simulink library "csu_gsh_gravity_spherical_harmonic_lib"  (R2014b)
settings: Solver=ode45  StartTime=0.0  StopTime=10.0  RelTol=1e-3
undefined symbols (not defined in the file or in its folder): central_body_flattening, gsh_a, gsh_b, gsh_c, gsh_deg, gsh_e, gsh_ep, gsh_n_degree, gsh_ord, gsh_s, magnitude
undefined symbols (not defined in the file): central_body_gravity_mu, central_body_radius
libraries: util_quat_lib x4, util_info_lib x2, util_common_lib x1
settings Model: Creator=mstewart  LastModifiedBy=mstewart

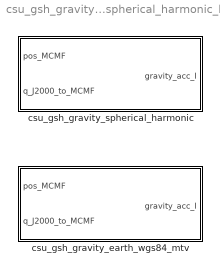
== system csu_gsh_gravity_spherical_harmonic_lib ==
  csu_gsh_gravity_earth_wgs84_mtv : Subsystem
  csu_gsh_gravity_spherical_harmonic : Subsystem  mask{mu_central_body=central_body_gravity_mu, r_central_body=central_body_radius}
      mask prompts: mu_central_body "Mu parameter for central body"; r_central_body "Radius of central body"

== system csu_gsh_gravity_spherical_harmonic_lib/csu_gsh_gravity_earth_wgs84_mtv ==
  pos_MCMF : Inport
  q_J2000_to_MCMF : Inport  Port=2
  Library Information : util_info_lib/Library Information  owner='NONE'
  earth_surface_gravity_with_j2 : Subsystem
  quaternion_conjugate : util_quat_lib/quaternion_conjugate  SystemSampleTime=-1
  quaternion_frame_transformation : util_quat_lib/quaternion_frame_transformation  SystemSampleTime=-1
  gravity_acc_I : Outport
  wires:
  earth_surface_gravity_with_j2/1(g_MCMF) -> quaternion_frame_transformation/1  "gravity_acc_MCMF"
  pos_MCMF/1 -> earth_surface_gravity_with_j2/1(pos_MCMF)
  quaternion_conjugate/1 -> quaternion_frame_transformation/2
  quaternion_frame_transformation/1 -> gravity_acc_I/1
  q_J2000_to_MCMF/1 -> quaternion_conjugate/1

== system csu_gsh_gravity_spherical_harmonic_lib/csu_gsh_gravity_spherical_harmonic ==
  pos_MCMF : Inport
  q_J2000_to_MCMF : Inport  Port=2
  Library Information : util_info_lib/Library Information  owner='NONE'
  Spherical Harmonic Gravity Model : Subsystem
      mask Display:
      | port_label('input',1,'pos\_MCMF','texmode','on')
      | port_label('output',1,'g\_MCMF','texmode','on')
      | disp('Spherical Harmonic Gravity Model')
      | color('blue')
      | text(0.05,0.02,'MoonEx',...
      |  	'HorizontalAlignment','Left',...
      | 	'VerticalAlignment','bottom')
  quaternion_conjugate : util_quat_lib/quaternion_conjugate  SystemSampleTime=-1
  quaternion_frame_transformation : util_quat_lib/quaternion_frame_transformation  SystemSampleTime=-1
  gravity_acc_I : Outport
  wires:
  Spherical Harmonic Gravity Model/1(g_MCMF) -> quaternion_frame_transformation/1  "gravity_acc_MCMF"
  pos_MCMF/1 -> Spherical Harmonic Gravity Model/1(pos_MCMF)
  quaternion_conjugate/1 -> quaternion_frame_transformation/2
  quaternion_frame_transformation/1 -> gravity_acc_I/1
  q_J2000_to_MCMF/1 -> quaternion_conjugate/1

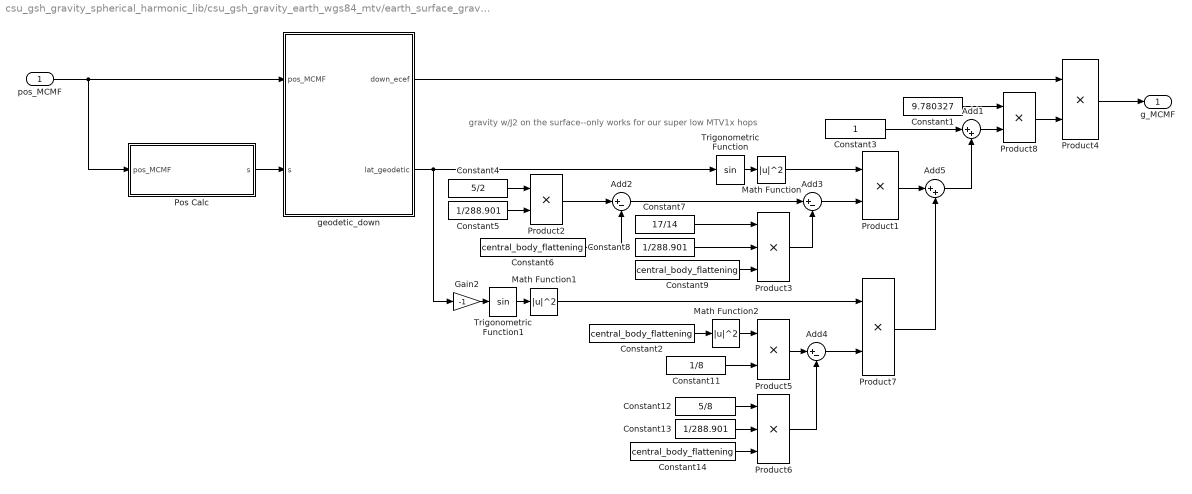
== system csu_gsh_gravity_spherical_harmonic_lib/csu_gsh_gravity_earth_wgs84_mtv/earth_surface_gravity_with_j2 ==
  note: gravity w/J2 on the surface--only works for our super low MTV1x hops
  pos_MCMF : Inport
  Add1 : Sum  Inputs=|++
  Add2 : Sum  Inputs=|+-
  Add3 : Sum  Inputs=|+-
  Add4 : Sum  Inputs=|+-
  Add5 : Sum  Inputs=|++
  Constant1 : Constant  Value=9.780327
  Constant11 : Constant  Value=1/8
  Constant12 : Constant  Value=5/8
  Constant13 : Constant  Value=1/288.901
  Constant{2,6,9,14} (4 alike) : Constant  Value=central_body_flattening
  Constant3 : Constant
  Constant4 : Constant  Value=5/2
  Constant5 : Constant  Value=1/288.901
  Constant7 : Constant  Value=17/14
  Constant8 : Constant  Value=1/288.901
  Gain2 : Gain  Gain=-1
  Math Function : Math  Operator=magnitude^2  SaturateOnIntegerOverflow=on
  Math Function1 : Math  Operator=magnitude^2  SaturateOnIntegerOverflow=on
  Math Function2 : Math  Operator=magnitude^2  SaturateOnIntegerOverflow=on
  Pos Calc : Subsystem
  Product{1..2,4..5,7..8} (6 alike) : Product
  Product3 : Product  Inputs=3
  Product6 : Product  Inputs=3
  Trigonometric Function : Trigonometry
  Trigonometric Function1 : Trigonometry
  geodetic_down : Subsystem
  g_MCMF : Outport
  wires:
  geodetic_down/1(down_ecef) -> Product4/1
  Product8/1 -> Product4/2
  Constant1/1 -> Product8/1
  Add1/1 -> Product8/2
  Add5/1 -> Add1/2
  Product7/1 -> Add5/2
  Product1/1 -> Add5/1
  Math Function1/1 -> Product7/1
  Add4/1 -> Product7/2
  Product6/1 -> Add4/2
  Product5/1 -> Add4/1
  Constant14/1 -> Product6/3
  Constant13/1 -> Product6/2
  Constant12/1 -> Product6/1
  Constant11/1 -> Product5/2
  Math Function2/1 -> Product5/1
  Constant2/1 -> Math Function2/1
  Add3/1 -> Product1/2
  Math Function/1 -> Product1/1
  Product3/1 -> Add3/2
  Add2/1 -> Add3/1
  Constant9/1 -> Product3/3
  Constant8/1 -> Product3/2
  Constant7/1 -> Product3/1
  Constant6/1 -> Add2/2
  Product2/1 -> Add2/1
  Constant5/1 -> Product2/2
  Constant4/1 -> Product2/1
  Gain2/1 -> Trigonometric Function1/1
  geodetic_down/2(lat_geodetic) -> Trigonometric Function/1, Gain2/1
  Trigonometric Function1/1 -> Math Function1/1
  Trigonometric Function/1 -> Math Function/1
  Constant3/1 -> Add1/1
  pos_MCMF/1 -> geodetic_down/1(pos_MCMF), Pos Calc/1(pos_MCMF)
  Pos Calc/1(s) -> geodetic_down/2(s)
  Product4/1 -> g_MCMF/1

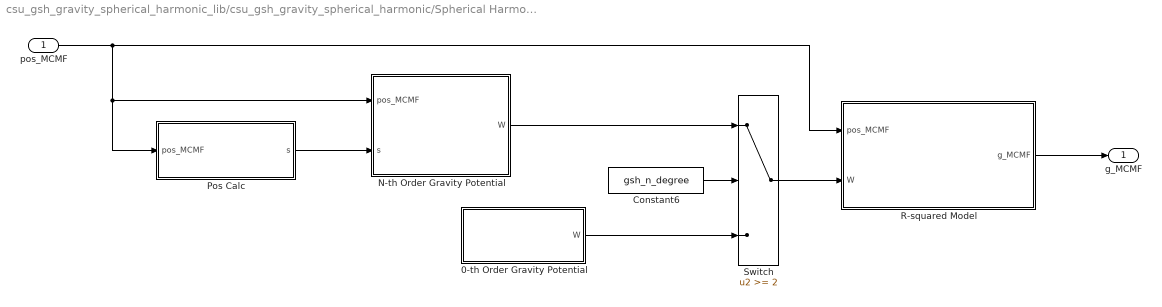
== system csu_gsh_gravity_spherical_harmonic_lib/csu_gsh_gravity_spherical_harmonic/Spherical Harmonic Gravity Model ==
  pos_MCMF : Inport
  0-th Order Gravity Potential : Subsystem
  Constant6 : Constant  Value=gsh_n_degree
  N-th Order Gravity Potential : Subsystem
  Pos Calc : Subsystem
  R-squared Model : Subsystem
  Switch : Switch  Threshold=2
  g_MCMF : Outport
  wires:
  pos_MCMF/1 -> R-squared Model/1(pos_MCMF), N-th Order Gravity Potential/1(pos_MCMF), Pos Calc/1(pos_MCMF)
  Switch/1 -> R-squared Model/2(W)
  Pos Calc/1(s) -> N-th Order Gravity Potential/2(s)
  0-th Order Gravity Potential/1(W) -> Switch/3
  N-th Order Gravity Potential/1(W) -> Switch/1
  Constant6/1 -> Switch/2
  R-squared Model/1(g_MCMF) -> g_MCMF/1

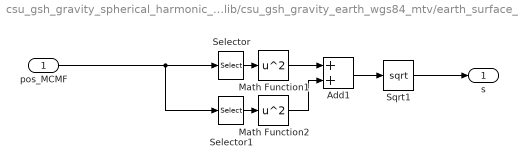
== system csu_gsh_gravity_spherical_harmonic_lib/csu_gsh_gravity_earth_wgs84_mtv/earth_surface_gravity_with_j2/Pos Calc ==
  pos_MCMF : Inport
  Add1 : Sum
  Math Function1 : Math  Operator=square  SaturateOnIntegerOverflow=on
  Math Function2 : Math  Operator=square  SaturateOnIntegerOverflow=on
  Selector : Selector  InputPortWidth=3  Indices=[1]
  Selector1 : Selector  InputPortWidth=3  Indices=[2]
  Sqrt1 : Sqrt  SaturateOnIntegerOverflow=on
  s : Outport
  wires:
  Math Function2/1 -> Add1/2
  Math Function1/1 -> Add1/1
  Sqrt1/1 -> s/1
  Add1/1 -> Sqrt1/1
  Selector1/1 -> Math Function2/1
  Selector/1 -> Math Function1/1
  pos_MCMF/1 -> Selector/1, Selector1/1

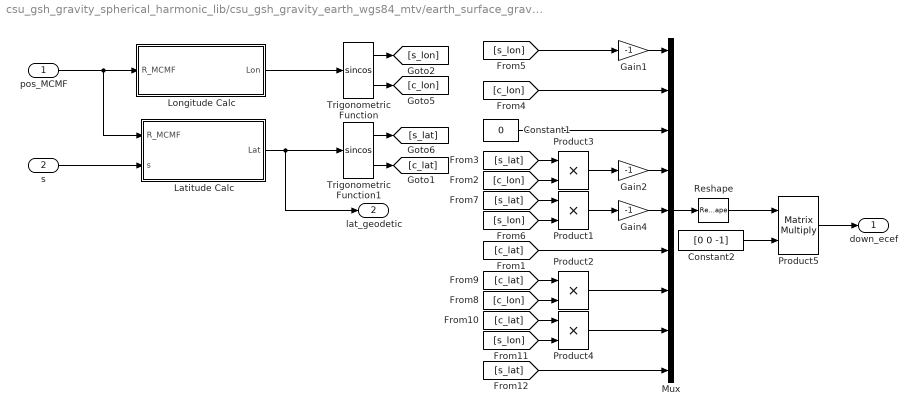
== system csu_gsh_gravity_spherical_harmonic_lib/csu_gsh_gravity_earth_wgs84_mtv/earth_surface_gravity_with_j2/geodetic_down ==
  pos_MCMF : Inport
  s : Inport  Port=2
  Constant1 : Constant  Value=0
  Constant2 : Constant  Value=[0 0 -1]
  Gain1 : Gain  Gain=-1
  Gain2 : Gain  Gain=-1
  Gain4 : Gain  Gain=-1
  Latitude Calc : Subsystem
  Longitude Calc : Subsystem
  Mux : Mux  Inputs=9
  Product{1..4} (4 alike) : Product  RndMeth=Zero
  Product5 : Product  Multiplication=Matrix(*)  RndMeth=Zero
  Reshape : Reshape  OutputDimensionality=Customize  OutputDimensions=[3,3]
  Trigonometric Function : Trigonometry  Operator=sincos
  Trigonometric Function1 : Trigonometry  Operator=sincos
  down_ecef : Outport
  lat_geodetic : Outport  Port=2
  wires:
  s/1 -> Latitude Calc/2(s)
  Product5/1 -> down_ecef/1
  Longitude Calc/1(Lon) -> Trigonometric Function/1
  Latitude Calc/1(Lat) -> Trigonometric Function1/1, lat_geodetic/1
  pos_MCMF/1 -> Longitude Calc/1(R_MCMF), Latitude Calc/1(R_MCMF)
  Trigonometric Function/1 -> [s_lon]
  Trigonometric Function/2 -> [c_lon]
  Trigonometric Function1/1 -> [s_lat]
  Trigonometric Function1/2 -> [c_lat]
  Gain1/1 -> Mux/1
  [s_lon] -> Gain1/1
  [c_lon] -> Mux/2
  Constant1/1 -> Mux/3
  [s_lat] -> Product3/1
  [c_lon] -> Product3/2
  Product3/1 -> Gain2/1
  Gain2/1 -> Mux/4
  [s_lat] -> Product1/1
  [s_lon] -> Product1/2
  Product1/1 -> Gain4/1
  Gain4/1 -> Mux/5
  [c_lat] -> Mux/6
  [c_lat] -> Product2/1
  Product2/1 -> Mux/7
  [c_lon] -> Product2/2
  [c_lat] -> Product4/1
  Product4/1 -> Mux/8
  [s_lon] -> Product4/2
  [s_lat] -> Mux/9
  Mux/1 -> Reshape/1
  Reshape/1 -> Product5/1
  Constant2/1 -> Product5/2

== system csu_gsh_gravity_spherical_harmonic_lib/csu_gsh_gravity_spherical_harmonic/Spherical Harmonic Gravity Model/0-th Order Gravity Potential ==
  Constant : Constant  Value=0
  W : Outport
  wires:
  Constant/1 -> W/1

== system csu_gsh_gravity_spherical_harmonic_lib/csu_gsh_gravity_spherical_harmonic/Spherical Harmonic Gravity Model/N-th Order Gravity Potential ==
  pos_MCMF : Inport
  s : Inport  Port=2
  Altitude Calc : Subsystem
  Gravity Potential : Subsystem
  Latitude Calc : Subsystem
  Longitude Calc : Subsystem
  W : Outport
  wires:
  s/1 -> Latitude Calc/2(s), Altitude Calc/2(s)
  Gravity Potential/1(W) -> W/1
  Longitude Calc/1(Lon) -> Gravity Potential/1(Lon)
  Altitude Calc/1(Alt) -> Gravity Potential/3(Alt)
  Latitude Calc/1(Lat) -> Altitude Calc/1(Lat), Gravity Potential/2(Lat)
  pos_MCMF/1 -> Longitude Calc/1(R_MCMF), Latitude Calc/1(R_MCMF)

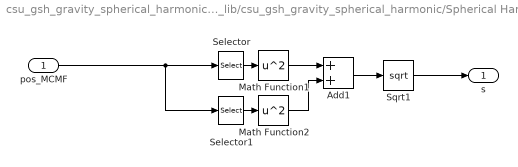
== system csu_gsh_gravity_spherical_harmonic_lib/csu_gsh_gravity_spherical_harmonic/Spherical Harmonic Gravity Model/Pos Calc ==
  pos_MCMF : Inport
  Add1 : Sum
  Math Function1 : Math  Operator=square  SaturateOnIntegerOverflow=on
  Math Function2 : Math  Operator=square  SaturateOnIntegerOverflow=on
  Selector : Selector  InputPortWidth=3  Indices=[1]
  Selector1 : Selector  InputPortWidth=3  Indices=[2]
  Sqrt1 : Sqrt  SaturateOnIntegerOverflow=on
  s : Outport
  wires:
  Math Function2/1 -> Add1/2
  Math Function1/1 -> Add1/1
  Sqrt1/1 -> s/1
  Add1/1 -> Sqrt1/1
  Selector1/1 -> Math Function2/1
  Selector/1 -> Math Function1/1
  pos_MCMF/1 -> Selector/1, Selector1/1

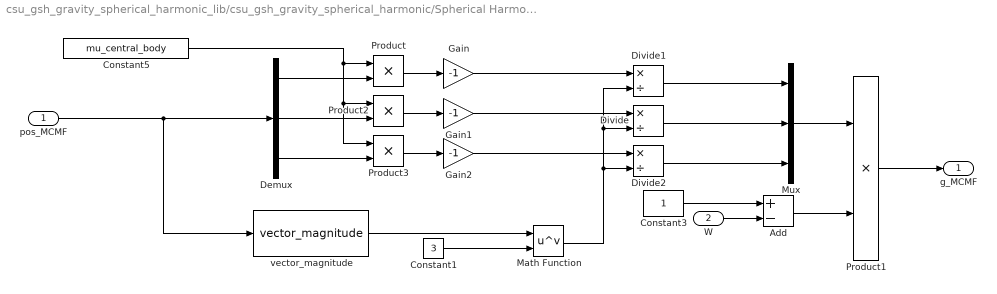
== system csu_gsh_gravity_spherical_harmonic_lib/csu_gsh_gravity_spherical_harmonic/Spherical Harmonic Gravity Model/R-squared Model ==
  pos_MCMF : Inport
  W : Inport  Port=2
  Add : Sum  Inputs=+-
  Constant1 : Constant  Value=3
  Constant3 : Constant
  Constant5 : Constant  Value=mu_central_body
  Demux : Demux  Outputs=3
  Divide : Product  Inputs=*/
  Divide1 : Product  Inputs=*/
  Divide2 : Product  Inputs=*/
  Gain : Gain  Gain=-1
  Gain1 : Gain  Gain=-1
  Gain2 : Gain  Gain=-1
  Math Function : Math  Operator=pow  SaturateOnIntegerOverflow=on
  Mux : Mux  Inputs=3
  Product : Product  RndMeth=Zero
  Product1 : Product
  Product2 : Product  RndMeth=Zero
  Product3 : Product  RndMeth=Zero
  vector_magnitude : util_common_lib/vector_magnitude  SystemSampleTime=-1
  g_MCMF : Outport
  wires:
  pos_MCMF/1 -> Demux/1, vector_magnitude/1
  Mux/1 -> Product1/1
  Constant1/1 -> Math Function/2
  Math Function/1 -> Divide2/2, Divide/2, Divide1/2
  vector_magnitude/1 -> Math Function/1
  Divide2/1 -> Mux/3
  Divide/1 -> Mux/2
  Divide1/1 -> Mux/1
  Gain2/1 -> Divide2/1
  Gain1/1 -> Divide/1
  Gain/1 -> Divide1/1
  Product/1 -> Gain/1
  Product2/1 -> Gain1/1
  Product3/1 -> Gain2/1
  Constant5/1 -> Product/1, Product2/1, Product3/1
  Demux/2 -> Product2/2
  Demux/1 -> Product/2
  Demux/3 -> Product3/2
  W/1 -> Add/2
  Add/1 -> Product1/2
  Constant3/1 -> Add/1
  Product1/1 -> g_MCMF/1

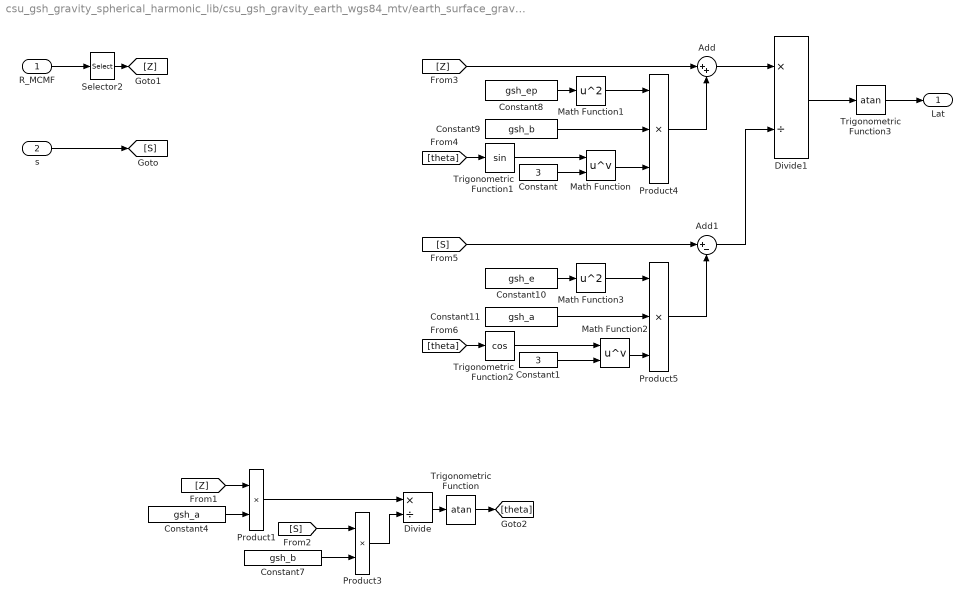
== system csu_gsh_gravity_spherical_harmonic_lib/csu_gsh_gravity_earth_wgs84_mtv/earth_surface_gravity_with_j2/geodetic_down/Latitude Calc ==
  R_MCMF : Inport
  s : Inport  Port=2
  Add : Sum  Inputs=|++
  Add1 : Sum  Inputs=|+-
  Constant : Constant  Value=3
  Constant1 : Constant  Value=3
  Constant10 : Constant  Value=gsh_e
  Constant11 : Constant  Value=gsh_a
  Constant4 : Constant  Value=gsh_a
  Constant7 : Constant  Value=gsh_b
  Constant8 : Constant  Value=gsh_ep
  Constant9 : Constant  Value=gsh_b
  Divide : Product  Inputs=*/
  Divide1 : Product  Inputs=*/
  Math Function : Math  Operator=pow  SaturateOnIntegerOverflow=on
  Math Function1 : Math  Operator=square  SaturateOnIntegerOverflow=on
  Math Function2 : Math  Operator=pow  SaturateOnIntegerOverflow=on
  Math Function3 : Math  Operator=square  SaturateOnIntegerOverflow=on
  Product1 : Product
  Product3 : Product
  Product4 : Product  Inputs=3
  Product5 : Product  Inputs=3
  Selector2 : Selector  InputPortWidth=3  Indices=[3]
  Trigonometric Function : Trigonometry  Operator=atan
  Trigonometric Function1 : Trigonometry
  Trigonometric Function2 : Trigonometry  Operator=cos
  Trigonometric Function3 : Trigonometry  Operator=atan
  Lat : Outport
  wires:
  [theta] -> Trigonometric Function2/1
  [theta] -> Trigonometric Function1/1
  Trigonometric Function/1 -> [theta]
  Trigonometric Function3/1 -> Lat/1
  Divide1/1 -> Trigonometric Function3/1
  Add1/1 -> Divide1/2
  Product5/1 -> Add1/2
  Math Function2/1 -> Product5/3
  Constant1/1 -> Math Function2/2
  Trigonometric Function2/1 -> Math Function2/1
  Constant11/1 -> Product5/2
  Math Function3/1 -> Product5/1
  Constant10/1 -> Math Function3/1
  [S] -> Add1/1
  Add/1 -> Divide1/1
  Product4/1 -> Add/2
  Math Function/1 -> Product4/3
  Constant/1 -> Math Function/2
  Trigonometric Function1/1 -> Math Function/1
  Constant9/1 -> Product4/2
  Math Function1/1 -> Product4/1
  Constant8/1 -> Math Function1/1
  [Z] -> Add/1
  Divide/1 -> Trigonometric Function/1
  Product3/1 -> Divide/2
  [S] -> Product3/1
  Constant7/1 -> Product3/2
  Product1/1 -> Divide/1
  [Z] -> Product1/1
  Constant4/1 -> Product1/2
  Selector2/1 -> [Z]
  s/1 -> [S]
  R_MCMF/1 -> Selector2/1

== system csu_gsh_gravity_spherical_harmonic_lib/csu_gsh_gravity_earth_wgs84_mtv/earth_surface_gravity_with_j2/geodetic_down/Longitude Calc ==
  R_MCMF : Inport
  Divide : Product  Inputs=*/
  Selector1 : Selector  InputPortWidth=3  Indices=[1]
  Selector2 : Selector  InputPortWidth=3  Indices=[2]
  Trigonometric Function : Trigonometry  Operator=atan
  Lon : Outport
  wires:
  Trigonometric Function/1 -> Lon/1
  Divide/1 -> Trigonometric Function/1
  Selector1/1 -> Divide/2
  Selector2/1 -> Divide/1
  R_MCMF/1 -> Selector2/1, Selector1/1

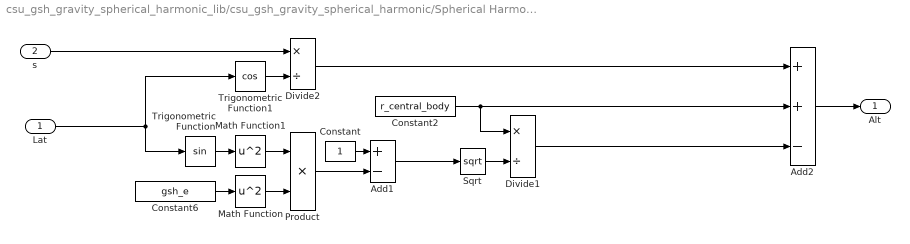
== system csu_gsh_gravity_spherical_harmonic_lib/csu_gsh_gravity_spherical_harmonic/Spherical Harmonic Gravity Model/N-th Order Gravity Potential/Altitude Calc ==
  Lat : Inport
  s : Inport  Port=2
  Add1 : Sum  Inputs=+-
  Add2 : Sum  Inputs=++-
  Constant : Constant
  Constant2 : Constant  Value=r_central_body
  Constant6 : Constant  Value=gsh_e
  Divide1 : Product  Inputs=*/
  Divide2 : Product  Inputs=*/
  Math Function : Math  Operator=square  SaturateOnIntegerOverflow=on
  Math Function1 : Math  Operator=square  SaturateOnIntegerOverflow=on
  Product : Product
  Sqrt : Sqrt  SaturateOnIntegerOverflow=on
  Trigonometric Function : Trigonometry
  Trigonometric Function1 : Trigonometry  Operator=cos
  Alt : Outport
  wires:
  Add2/1 -> Alt/1
  Trigonometric Function1/1 -> Divide2/2
  s/1 -> Divide2/1
  Lat/1 -> Trigonometric Function1/1, Trigonometric Function/1
  Divide1/1 -> Add2/3
  Divide2/1 -> Add2/1
  Add1/1 -> Sqrt/1
  Product/1 -> Add1/2
  Constant/1 -> Add1/1
  Math Function1/1 -> Product/1
  Trigonometric Function/1 -> Math Function1/1
  Math Function/1 -> Product/2
  Sqrt/1 -> Divide1/2
  Constant2/1 -> Divide1/1, Add2/2
  Constant6/1 -> Math Function/1

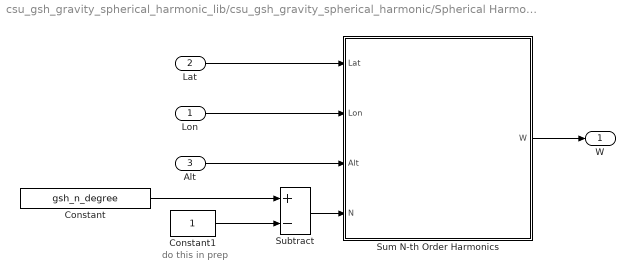
== system csu_gsh_gravity_spherical_harmonic_lib/csu_gsh_gravity_spherical_harmonic/Spherical Harmonic Gravity Model/N-th Order Gravity Potential/Gravity Potential ==
  note: do this in prep
  Lon : Inport
  Lat : Inport  Port=2
  Alt : Inport  Port=3
  Constant : Constant  Value=gsh_n_degree
  Constant1 : Constant
  Subtract : Sum  Inputs=+-
  Sum N-th Order Harmonics : Subsystem  TreatAsAtomicUnit=on
  W : Outport
  wires:
  Sum N-th Order Harmonics/1(W) -> W/1
  Subtract/1 -> Sum N-th Order Harmonics/4(N)
  Alt/1 -> Sum N-th Order Harmonics/3(Alt)
  Lon/1 -> Sum N-th Order Harmonics/2(Lon)
  Lat/1 -> Sum N-th Order Harmonics/1(Lat)
  Constant/1 -> Subtract/1
  Constant1/1 -> Subtract/2

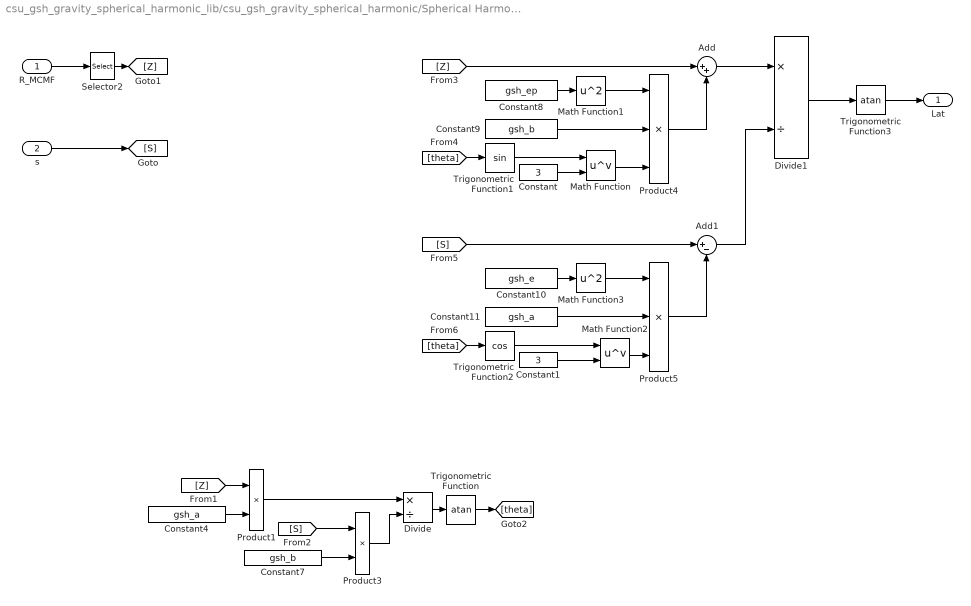
== system csu_gsh_gravity_spherical_harmonic_lib/csu_gsh_gravity_spherical_harmonic/Spherical Harmonic Gravity Model/N-th Order Gravity Potential/Latitude Calc ==
  R_MCMF : Inport
  s : Inport  Port=2
  Add : Sum  Inputs=|++
  Add1 : Sum  Inputs=|+-
  Constant : Constant  Value=3
  Constant1 : Constant  Value=3
  Constant10 : Constant  Value=gsh_e
  Constant11 : Constant  Value=gsh_a
  Constant4 : Constant  Value=gsh_a
  Constant7 : Constant  Value=gsh_b
  Constant8 : Constant  Value=gsh_ep
  Constant9 : Constant  Value=gsh_b
  Divide : Product  Inputs=*/
  Divide1 : Product  Inputs=*/
  Math Function : Math  Operator=pow  SaturateOnIntegerOverflow=on
  Math Function1 : Math  Operator=square  SaturateOnIntegerOverflow=on
  Math Function2 : Math  Operator=pow  SaturateOnIntegerOverflow=on
  Math Function3 : Math  Operator=square  SaturateOnIntegerOverflow=on
  Product1 : Product
  Product3 : Product
  Product4 : Product  Inputs=3
  Product5 : Product  Inputs=3
  Selector2 : Selector  InputPortWidth=3  Indices=[3]
  Trigonometric Function : Trigonometry  Operator=atan
  Trigonometric Function1 : Trigonometry
  Trigonometric Function2 : Trigonometry  Operator=cos
  Trigonometric Function3 : Trigonometry  Operator=atan
  Lat : Outport
  wires:
  [theta] -> Trigonometric Function2/1
  [theta] -> Trigonometric Function1/1
  Trigonometric Function/1 -> [theta]
  Trigonometric Function3/1 -> Lat/1
  Divide1/1 -> Trigonometric Function3/1
  Add1/1 -> Divide1/2
  Product5/1 -> Add1/2
  Math Function2/1 -> Product5/3
  Constant1/1 -> Math Function2/2
  Trigonometric Function2/1 -> Math Function2/1
  Constant11/1 -> Product5/2
  Math Function3/1 -> Product5/1
  Constant10/1 -> Math Function3/1
  [S] -> Add1/1
  Add/1 -> Divide1/1
  Product4/1 -> Add/2
  Math Function/1 -> Product4/3
  Constant/1 -> Math Function/2
  Trigonometric Function1/1 -> Math Function/1
  Constant9/1 -> Product4/2
  Math Function1/1 -> Product4/1
  Constant8/1 -> Math Function1/1
  [Z] -> Add/1
  Divide/1 -> Trigonometric Function/1
  Product3/1 -> Divide/2
  [S] -> Product3/1
  Constant7/1 -> Product3/2
  Product1/1 -> Divide/1
  [Z] -> Product1/1
  Constant4/1 -> Product1/2
  Selector2/1 -> [Z]
  s/1 -> [S]
  R_MCMF/1 -> Selector2/1

== system csu_gsh_gravity_spherical_harmonic_lib/csu_gsh_gravity_spherical_harmonic/Spherical Harmonic Gravity Model/N-th Order Gravity Potential/Longitude Calc ==
  R_MCMF : Inport
  Divide : Product  Inputs=*/
  Selector1 : Selector  InputPortWidth=3  Indices=[1]
  Selector2 : Selector  InputPortWidth=3  Indices=[2]
  Trigonometric Function : Trigonometry  Operator=atan
  Lon : Outport
  wires:
  Trigonometric Function/1 -> Lon/1
  Divide/1 -> Trigonometric Function/1
  Selector1/1 -> Divide/2
  Selector2/1 -> Divide/1
  R_MCMF/1 -> Selector2/1, Selector1/1

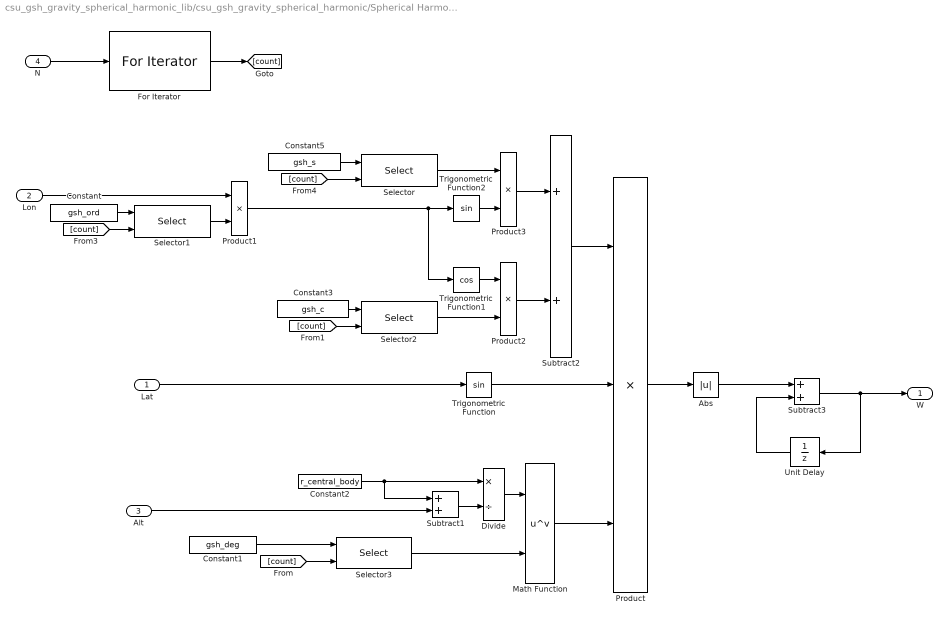
== system csu_gsh_gravity_spherical_harmonic_lib/csu_gsh_gravity_spherical_harmonic/Spherical Harmonic Gravity Model/N-th Order Gravity Potential/Gravity Potential/Sum N-th Order Harmonics ==
  Lat : Inport
  Lon : Inport  Port=2
  Alt : Inport  Port=3
  N : Inport  Port=4
  Abs : Abs
  Constant : Constant  Value=gsh_ord
  Constant1 : Constant  Value=gsh_deg
  Constant2 : Constant  Value=r_central_body
  Constant3 : Constant  Value=gsh_c
  Constant5 : Constant  Value=gsh_s
  Divide : Product  Inputs=*/
  For Iterator : ForIterator  ResetStates=reset  IterationSource=external
  Math Function : Math  Operator=pow  SaturateOnIntegerOverflow=on
  Product : Product  Inputs=3
  Product1 : Product
  Product2 : Product
  Product3 : Product
  Selector{,1..3} (4 alike) : Selector  InputPortWidth=gsh_n_degree-1  IndexOptions=Index vector (port)  Indices=[1 3]
  Subtract1 : Sum
  Subtract2 : Sum
  Subtract3 : Sum
  Trigonometric Function : Trigonometry
  Trigonometric Function1 : Trigonometry  Operator=cos
  Trigonometric Function2 : Trigonometry
  Unit Delay : UnitDelay  SampleTime=-1
  W : Outport
  wires:
  Unit Delay/1 -> Subtract3/2
  Abs/1 -> Subtract3/1
  N/1 -> For Iterator/1
  Subtract3/1 -> Unit Delay/1, W/1
  For Iterator/1 -> [count]
  Product/1 -> Abs/1
  Subtract2/1 -> Product/1
  Trigonometric Function/1 -> Product/2
  Product3/1 -> Subtract2/1
  Selector/1 -> Product3/1
  Trigonometric Function2/1 -> Product3/2
  Product1/1 -> Trigonometric Function2/1, Trigonometric Function1/1
  Product2/1 -> Subtract2/2
  Selector2/1 -> Product2/2
  Trigonometric Function1/1 -> Product2/1
  [count] -> Selector/2
  Constant5/1 -> Selector/1
  Lon/1 -> Product1/1
  Selector1/1 -> Product1/2
  [count] -> Selector1/2
  Constant/1 -> Selector1/1
  [count] -> Selector2/2
  Constant3/1 -> Selector2/1
  Math Function/1 -> Product/3
  Lat/1 -> Trigonometric Function/1
  Selector3/1 -> Math Function/2
  [count] -> Selector3/2
  Constant1/1 -> Selector3/1
  Divide/1 -> Math Function/1
  Subtract1/1 -> Divide/2
  Alt/1 -> Subtract1/2
  Constant2/1 -> Divide/1, Subtract1/1
